simulink model "FM"  (R2020a)
settings: Solver=VariableStepAuto  StartTime=0.0  StopTime=10.0  MaxStep=1e-3  RelTol=1e-3
settings Model: Creator=a1  LastModifiedBy=a1

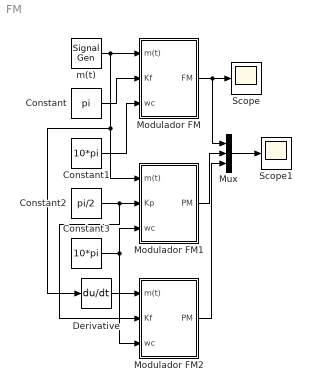
== system FM ==
  Constant : Constant  Value=pi
  Constant1 : Constant  Value=10*pi
  Constant2 : Constant  Value=pi/2
  Constant3 : Constant  Value=10*pi
  Derivative : Derivative
  Modulador FM : Subsystem
  Modulador FM1 : Subsystem
  Modulador FM2 : Subsystem
  Mux : Mux  Inputs=3
  Scope : Scope
  Scope1 : Scope
  m(t) : SignalGenerator  Units=rad/sec
  wires:
  m(t)/1 -> Derivative/1, Modulador FM1/1(m(t)), Modulador FM/1(m(t))
  Constant/1 -> Modulador FM/2(Kf)
  Constant1/1 -> Modulador FM/3(wc)
  Modulador FM/1(FM) -> Mux/1, Scope/1
  Constant2/1 -> Modulador FM2/2(Kf), Modulador FM1/2(Kp)
  Constant3/1 -> Modulador FM2/3(wc), Modulador FM1/3(wc)
  Mux/1 -> Scope1/1
  Modulador FM1/1(PM) -> Mux/2
  Derivative/1 -> Modulador FM2/1(m(t))
  Modulador FM2/1(PM) -> Mux/3

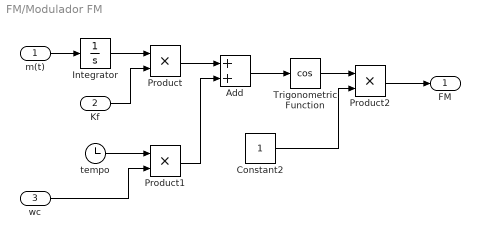
== system FM/Modulador FM ==
  m(t) : Inport
  Kf : Inport  Port=2
  wc : Inport  Port=3
  Add : Sum
  Constant2 : Constant
  Integrator : Integrator
  Product : Product
  Product1 : Product
  Product2 : Product
  Trigonometric Function : Trigonometry  Operator=cos
  tempo : Clock
  FM : Outport
  wires:
  Product2/1 -> FM/1
  Product1/1 -> Add/2
  Kf/1 -> Product/2
  Product/1 -> Add/1
  Trigonometric Function/1 -> Product2/1
  m(t)/1 -> Integrator/1
  Constant2/1 -> Product2/2
  Integrator/1 -> Product/1
  wc/1 -> Product1/2
  Add/1 -> Trigonometric Function/1
  tempo/1 -> Product1/1

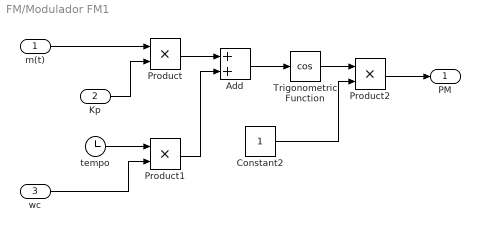
== system FM/Modulador FM1 ==
  m(t) : Inport
  Kp : Inport  Port=2
  wc : Inport  Port=3
  Add : Sum
  Constant2 : Constant
  Product : Product
  Product1 : Product
  Product2 : Product
  Trigonometric Function : Trigonometry  Operator=cos
  tempo : Clock
  PM : Outport
  wires:
  Product2/1 -> PM/1
  Product1/1 -> Add/2
  Kp/1 -> Product/2
  Product/1 -> Add/1
  Trigonometric Function/1 -> Product2/1
  Constant2/1 -> Product2/2
  m(t)/1 -> Product/1
  wc/1 -> Product1/2
  Add/1 -> Trigonometric Function/1
  tempo/1 -> Product1/1

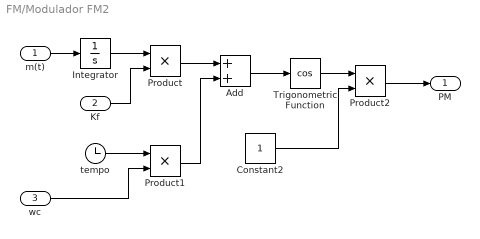
== system FM/Modulador FM2 ==
  m(t) : Inport
  Kf : Inport  Port=2
  wc : Inport  Port=3
  Add : Sum
  Constant2 : Constant
  Integrator : Integrator
  Product : Product
  Product1 : Product
  Product2 : Product
  Trigonometric Function : Trigonometry  Operator=cos
  tempo : Clock
  PM : Outport
  wires:
  Product2/1 -> PM/1
  Product1/1 -> Add/2
  Kf/1 -> Product/2
  Product/1 -> Add/1
  Trigonometric Function/1 -> Product2/1
  m(t)/1 -> Integrator/1
  Constant2/1 -> Product2/2
  Integrator/1 -> Product/1
  wc/1 -> Product1/2
  Add/1 -> Trigonometric Function/1
  tempo/1 -> Product1/1
